simulink model "MassSPDamper"  (R2020a)
settings: Solver=VariableStepAuto  StartTime=0.0  StopTime=10.0  MaxStep=1e-3  RelTol=1e-3
values from neighbouring files (symbols this model uses):
  b = 10    [run_model_script.m]
  k = 400    [run_model_script.m]
  m = diff_val_mass(i)    [run_model_script.m]
undefined symbols (not defined in the file or in its folder): x
settings Model: Creator=Administrator  LastModifiedBy=Administrator

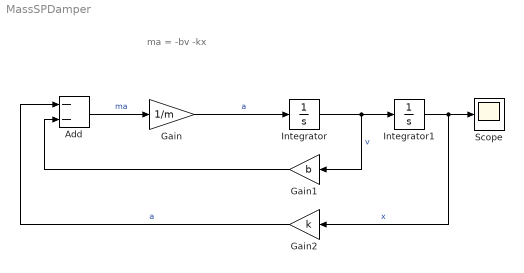
== system MassSPDamper ==
  note: ma = -bv -kx
  Add : Sum  Inputs=--
  Gain : Gain  Gain=1/m
  Gain1 : Gain  Gain=b
  Gain2 : Gain  Gain=k
  Integrator : Integrator
  Integrator1 : Integrator  InitialCondition=x
  Scope : Scope
  wires:
  Gain/1 -> Integrator/1  "a"
  Add/1 -> Gain/1  "ma"
  Integrator/1 -> Gain1/1, Integrator1/1  "v"
  Integrator1/1 -> Scope/1, Gain2/1  "x"
  Gain1/1 -> Add/2
  Gain2/1 -> Add/1  "a"
